simulink model "three_phase_fb_inverter"  (Simulink 6.1)
settings: Solver=ode23tb  StartTime=0.0  StopTime=0.1499  MaxStep=5e-5  RelTol=1e-3  AbsTol=.01
libraries: powerlib x17
settings Model: LastModifiedBy=ThinkPad
settings DebuggingCC: SolverPrmCheckMsg=warning

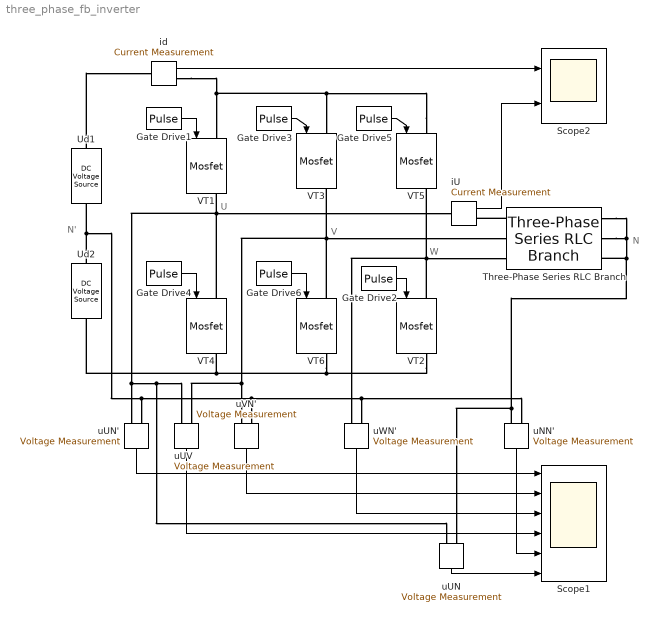
== system three_phase_fb_inverter ==
  note: N'
  note: N
  note: U
  note: V
  note: W
  Gate Drive1 : DiscretePulseGenerator  PulseType=Time based  Period=0.02  PulseWidth=49.5
  Gate Drive2 : DiscretePulseGenerator  PulseType=Time based  Period=0.02  PulseWidth=49.5  PhaseDelay=0.00333
  Gate Drive3 : DiscretePulseGenerator  PulseType=Time based  Period=0.02  PulseWidth=49.5  PhaseDelay=0.00667
  Gate Drive4 : DiscretePulseGenerator  PulseType=Time based  Period=0.02  PulseWidth=49.5  PhaseDelay=0.01
  Gate Drive5 : DiscretePulseGenerator  PulseType=Time based  Period=0.02  PulseWidth=49.5  PhaseDelay=0.01333
  Gate Drive6 : DiscretePulseGenerator  PulseType=Time based  Period=0.02  PulseWidth=49.5  PhaseDelay=0.01667
  Scope1 : Scope  NumInputPorts=6
      settings: TimeRange=0.05  YMin=-200~-200~-200~-300~-200~-200  YMax=200~200~200~300~200~200  SampleTime=2e-4
  Scope2 : Scope  NumInputPorts=2
      settings: TimeRange=0.05  YMin=-20~-20  YMax=20~20  SampleTime=2e-4
  Three-Phase Series RLC Branch : powerlib/Elements/Three-Phase Series RLC Branch  PhysicalDomain=powersysdomain  SubClassName=unknown  LeftPortType=p1  RightPortType=p1  LConnTagsString=A|B|C  RConnTagsString=A|B|C  Resistance=10  Inductance=0.02  Capacitance=inf  Measurements=Branch voltages and currents
  Ud1 : powerlib/Electrical Sources/DC Voltage Source  Orientation=up  Amplitude=100  Measurements=None
  Ud2 : powerlib/Electrical Sources/DC Voltage Source  Orientation=up  Amplitude=100  Measurements=None
  VT{1..6} (6 alike) : powerlib/Power Electronics/Mosfet  Orientation=down  Ron=0.01  Lon=1e-7  Rd=.01  IC=0  Rs=5  Cs=1e-6  Measurements=on
  iU : powerlib/Measurements/Current Measurement  PhasorSimulation=off  OutputType=Complex  PSBequivalent=0
  id : powerlib/Measurements/Current Measurement  PhasorSimulation=off  OutputType=Complex  PSBequivalent=0
  uNN' : powerlib/Measurements/Voltage Measurement  Orientation=down  PhasorSimulation=off  OutputType=Complex  PSBequivalent=0
  uUN : powerlib/Measurements/Voltage Measurement  Orientation=down  PhasorSimulation=off  OutputType=Complex  PSBequivalent=0
  uUN' : powerlib/Measurements/Voltage Measurement  Orientation=down  PhasorSimulation=off  OutputType=Complex  PSBequivalent=0
  uUV : powerlib/Measurements/Voltage Measurement  Orientation=down  PhasorSimulation=off  OutputType=Complex  PSBequivalent=0
  uVN' : powerlib/Measurements/Voltage Measurement  Orientation=down  PhasorSimulation=off  OutputType=Complex  PSBequivalent=0
  uWN' : powerlib/Measurements/Voltage Measurement  Orientation=down  PhasorSimulation=off  OutputType=Complex  PSBequivalent=0
  wires:
  Gate Drive1/1 -> VT1/1
  Gate Drive4/1 -> VT4/1
  Gate Drive3/1 -> VT3/1
  Gate Drive6/1 -> VT6/1
  Gate Drive5/1 -> VT5/1
  Gate Drive2/1 -> VT2/1
  uUN'/1 -> Scope1/1
  uVN'/1 -> Scope1/2
  uWN'/1 -> Scope1/3
  uUV/1 -> Scope1/4
  uNN'/1 -> Scope1/5
  id/1 -> Scope2/1
  iU/1 -> Scope2/2
  uUN/1 -> Scope1/6
  connections:
  VT3/RConn1 -- VT6/LConn1 -- Three-Phase Series RLC Branch/LConn2 -- uVN'/LConn1 -- uUV/LConn2
  VT1/RConn1 -- VT4/LConn1 -- iU/LConn1 -- uUN'/LConn1 -- uUV/LConn1 -- uUN/LConn1
  VT2/RConn1 -- VT6/RConn1 -- VT4/RConn1 -- Ud2/LConn1
  VT5/LConn1 -- VT3/LConn1 -- VT1/LConn1 -- id/RConn1
  VT5/RConn1 -- VT2/LConn1 -- Three-Phase Series RLC Branch/LConn3 -- uWN'/LConn1
  Ud2/RConn1 -- Ud1/LConn1 -- uUN'/LConn2 -- uVN'/LConn2 -- uWN'/LConn2 -- uNN'/LConn2
  uNN'/LConn1 -- Three-Phase Series RLC Branch/RConn1 -- Three-Phase Series RLC Branch/RConn2 -- Three-Phase Series RLC Branch/RConn3 -- uUN/LConn2
  Ud1/RConn1 -- id/LConn1
  Three-Phase Series RLC Branch/LConn1 -- iU/RConn1
